simulink model "thermo_simple_with_imc"  (R2017b)
settings: Solver=ode4  StartTime=0.0  StopTime=t_sim  FixedStep=Ts  RelTol=1e-3  EnableMultiTasking=on
undefined symbols (not defined in the file or in its folder): baud, com, D, fTf, fTl, fTt, I, input_fan, input_lamp, input_led, K0, P, reg_output, reg_regulate, reg_request, reg_type, T0, Tf, Ts, Umax, Umin, vstupy, vystupy
libraries: simulink x1, tos_lib x1
settings Model: Creator=tom  LastModifiedBy=www-data
settings DataIOCC: SaveFormat=Array  SignalLoggingSaveFormat=ModelDataLogs  SaveOutput=off  SignalLogging=off  SaveTime=off
settings OptimizationCC: ExpressionDepthLimit=2147483647  LifeSpan=inf
settings DebuggingCC: AlgebraicLoopMsg=none  ArtificialAlgebraicLoopMsg=none  UnderspecifiedInitializationDetection=Classic  MergeDetectMultiDrivingBlocksExec=none  SolverPrmCheckMsg=warning  FcnCallInpInsideContextMsg=warning  StateNameClashWarn=warning  StrictBusMsg=Warning  SFUnexpectedBacktrackingDiag=warning  SFNoUnconditionalDefaultTransitionDiag=warning  SFExecutionAtInitializationDiag=none
settings HardwareCC: ProdBitPerPointer=32  ProdBitPerSizeT=32  ProdBitPerPtrDiffT=32  ProdLargestAtomicFloat=None  ProdIntDivRoundTo=Undefined  ProdEndianess=Unspecified  ProdWordSize=32  ProdHWDeviceType=32-bit Generic
settings ModelReferenceCC: PropagateSignalLabelsOutOfModel=off
settings CodeAppCC: StateflowObjectComments=on
settings GRTTargetCC: TargetLangStandard=C89/C90 (ANSI)  GeneratePreprocessorConditionals=Disable all  CombineOutputUpdateFcns=off  GRTInterface=on
settings ConfigComp: CovMetricSettings=dw  CovHtmlReporting=on  CovSaveCumulativeToWorkspaceVar=on  CovSaveSingleToWorkspaceVar=on  CovExternalEMLEnable=off  CovSFcnEnable=off

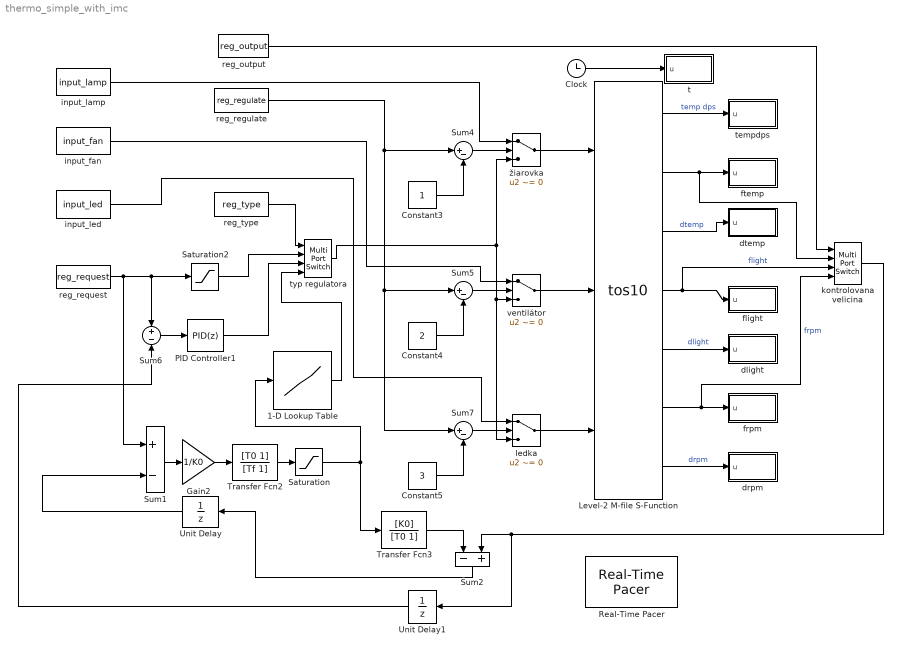
== system thermo_simple_with_imc ==
  1-D Lookup Table : Lookup_n-D  NumberOfTableDimensions=1  BreakpointsForDimension1=vystupy  Table=vstupy  UseLastTableValue=on  InputSameDT=on
  Clock : Clock
  Constant3 : Constant  SampleTime=Ts
  Constant4 : Constant  Value=2  SampleTime=Ts
  Constant5 : Constant  Value=3  SampleTime=Ts
  Gain2 : Gain  Gain=1/K0  SaturateOnIntegerOverflow=on  OutDataTypeStr=Inherit: Same as input  ParamDataTypeStr=Inherit: Same as input
  Level-2 M-file S-Function : M-S-Function  FunctionName=tos10  Parameters=Ts,com,baud,fTt,fTl,fTf
  PID Controller1 : simulink/Continuous/PID Controller  Controller=PID  TimeDomain=Discrete-time  SampleTime=Ts  IntegratorMethod=Forward Euler  FilterMethod=Forward Euler  Form=Parallel  UseFilter=on  ControllerParametersSource=internal  P=P  I=I  D=D  N=10  InitialConditionSource=internal  InitialConditionForIntegrator=0  InitialConditionForFilter=0  ExternalReset=none  LimitOutput=on  UpperSaturationLimit=100  LowerSaturationLimit=0  LinearizeAsGain=off  AntiWindupMode=clamping  Kb=10  TrackingMode=off  Kt=1  PParamMin=[]  PParamMax=[]  IParamMin=[]  IParamMax=[]  DParamMin=[]  DParamMax=[]  NParamMin=[]  NParamMax=[]  KbParamMin=[]  KbParamMax=[]  KtParamMin=[]  KtParamMax=[]  POutMin=[]  POutMax=[]  IOutMin=[]  IOutMax=[]  DOutMin=[]  DOutMax=[]  NOutMin=[]  NOutMax=[]  KbOutMin=[]  KbOutMax=[]  KtOutMin=[]  KtOutMax=[]  IntegratorOutMin=[]  IntegratorOutMax=[]  FilterOutMin=[]  FilterOutMax=[]  SumOutMin=[]  SumOutMax=[]  SumI1OutMin=[]  SumI1OutMax=[]  SumI1OutDataTypeStr=single  SumI2OutMin=[]  SumI2OutMax=[]  SumI3OutMin=[]  SumI3OutMax=[]  SumDOutMin=[]  SumDOutMax=[]  SaturationOutMin=[]  SaturationOutMax=[]  IntegratorContinuousStateAttributes=''  IntegratorStateMustResolveToSignalObject=off  IntegratorRTWStateStorageClass=Auto  FilterContinuousStateAttributes=''  FilterStateMustResolveToSignalObject=off  FilterRTWStateStorageClass=Auto  DifferentiatorICPrevScaledInput=0  DifferentiatorOutMin=[]  DifferentiatorOutMax=[]  InitialConditionSetting=State (most efficient)  FilterDiffOutCoefMin=[]  FilterDiffOutCoefMax=[]  SumDenOutMin=[]  SumDenOutMax=[]  SumNumOutMin=[]  SumNumOutMax=[]  ReciprocalOutMin=[]  ReciprocalOutMax=[]  DivideOutMin=[]  DivideOutMax=[]  TunerSelectOption=Transfer Function Based (PID Tuner App)
  Real-Time Pacer : tos_lib/Real-Time Pacer  simTimePerRealTime=1
  Saturation : Saturate  UpperLimit=Umax  LowerLimit=Umin
  Saturation2 : Saturate  UpperLimit=100  LowerLimit=0  SampleTime=Ts
  Sum1 : Sum  Inputs=+-  SaturateOnIntegerOverflow=on  InputSameDT=on  OutDataTypeStr=Inherit: Same as first input
  Sum2 : Sum  Inputs=-+  SaturateOnIntegerOverflow=on  InputSameDT=on  OutDataTypeStr=Inherit: Same as first input
  Sum4 : Sum  Inputs=|+-  SampleTime=Ts
  Sum5 : Sum  Inputs=|+-  SampleTime=Ts
  Sum6 : Sum  Inputs=+|-  SampleTime=Ts
  Sum7 : Sum  Inputs=|+-  SampleTime=Ts
  Transfer Fcn2 : TransferFcn  Numerator=[T0 1]  Denominator=[Tf 1]
  Transfer Fcn3 : TransferFcn  Numerator=[K0]  Denominator=[T0 1]
  Unit Delay : UnitDelay  SampleTime=-1
  Unit Delay1 : UnitDelay  SampleTime=Ts
  dlight : MATLAB Function  TreatAsAtomicUnit=on  SystemSampleTime=Ts
  drpm : MATLAB Function  TreatAsAtomicUnit=on  SystemSampleTime=Ts
  dtemp : MATLAB Function  TreatAsAtomicUnit=on  SystemSampleTime=Ts
  flight : MATLAB Function  TreatAsAtomicUnit=on  SystemSampleTime=Ts
  frpm : MATLAB Function  TreatAsAtomicUnit=on  SystemSampleTime=Ts
  ftemp : MATLAB Function  TreatAsAtomicUnit=on  SystemSampleTime=Ts
  input_fan : Constant  Value=input_fan  SampleTime=Ts
  input_lamp : Constant  Value=input_lamp  SampleTime=Ts
  input_led : Constant  Value=input_led  SampleTime=Ts
  kontrolovana velicina : MultiPortSwitch  OutDataTypeStr=double  SampleTime=Ts
  ledka : Switch  Criteria=u2 ~= 0  OutDataTypeStr=double
  reg_output : Constant  Value=reg_output  SampleTime=Ts
  reg_regulate : Constant  Value=reg_regulate  SampleTime=Ts
  reg_request : Constant  Value=reg_request  SampleTime=Ts
  reg_type : Constant  Value=reg_type  SampleTime=Ts
  t : MATLAB Function  TreatAsAtomicUnit=on  SystemSampleTime=Ts
  tempdps : MATLAB Function  TreatAsAtomicUnit=on  SystemSampleTime=Ts
  typ regulatora : MultiPortSwitch  OutDataTypeStr=double  SampleTime=Ts
  ventilátor : Switch  Criteria=u2 ~= 0  OutDataTypeStr=double
  žiarovka : Switch  Criteria=u2 ~= 0  OutDataTypeStr=double
  wires:
  ledka/1 -> Level-2 M-file S-Function/3
  Level-2 M-file S-Function/7 -> drpm/1(u)  "drpm"
  Sum4/1 -> žiarovka/2
  input_fan/1 -> ventilátor/1
  reg_regulate/1 -> Sum7/1, Sum5/1, Sum4/1
  Saturation2/1 -> typ regulatora/2
  Sum6/1 -> PID Controller1/1
  Level-2 M-file S-Function/1 -> tempdps/1(u)  "temp dps"
  Level-2 M-file S-Function/5 -> dlight/1(u)  "dlight"
  PID Controller1/1 -> typ regulatora/3
  žiarovka/1 -> Level-2 M-file S-Function/1
  ventilátor/1 -> Level-2 M-file S-Function/2
  reg_request/1 -> Sum1/1, Sum6/1, Saturation2/1
  Unit Delay1/1 -> Sum6/2
  Level-2 M-file S-Function/3 -> dtemp/1(u)  "dtemp"
  Constant4/1 -> Sum5/2
  Level-2 M-file S-Function/4 -> kontrolovana velicina/3, flight/1(u)  "flight"
  Level-2 M-file S-Function/6 -> kontrolovana velicina/4, frpm/1(u)  "frpm"
  Constant3/1 -> Sum4/2
  typ regulatora/1 -> žiarovka/3, ventilátor/3, ledka/3
  Clock/1 -> t/1(u)
  input_lamp/1 -> žiarovka/1
  reg_output/1 -> kontrolovana velicina/1
  Sum5/1 -> ventilátor/2
  Constant5/1 -> Sum7/2
  reg_type/1 -> typ regulatora/1
  kontrolovana velicina/1 -> Sum2/2, Unit Delay1/1
  Level-2 M-file S-Function/2 -> kontrolovana velicina/2, ftemp/1(u)
  Sum7/1 -> ledka/2
  input_led/1 -> ledka/1
  Saturation/1 -> 1-D Lookup Table/1, Transfer Fcn3/1
  Gain2/1 -> Transfer Fcn2/1
  Sum1/1 -> Gain2/1
  Transfer Fcn2/1 -> Saturation/1
  Transfer Fcn3/1 -> Sum2/1
  Unit Delay/1 -> Sum1/2
  Sum2/1 -> Unit Delay/1
  1-D Lookup Table/1 -> typ regulatora/4

== matlab function thermo_simple_with_imc/ftemp ==
  data: u input
function fcn(u)
%#eml
eml.extrinsic('num2str');
eml.extrinsic('strcat');
eml.extrinsic('evalin');
evalin('base',strcat('ftemp(end+1)=', num2str(u),';'));
end

== matlab function thermo_simple_with_imc/tempdps ==
  data: u input
function fcn(u)
%#eml
eml.extrinsic('num2str');
eml.extrinsic('strcat');
eml.extrinsic('evalin');
evalin('base',strcat('tempdps(end+1)=', num2str(u),';'));
end

== matlab function thermo_simple_with_imc/dtemp ==
  data: u input
function fcn(u)
%#eml
eml.extrinsic('num2str');
eml.extrinsic('strcat');
eml.extrinsic('evalin');
evalin('base',strcat('dtemp(end+1)=', num2str(u),';'));
end

== matlab function thermo_simple_with_imc/frpm ==
  data: u input
function fcn(u)
%#eml
eml.extrinsic('num2str');
eml.extrinsic('strcat');
eml.extrinsic('evalin');
evalin('base',strcat('frpm(end+1)=', num2str(u),';'));
end

== matlab function thermo_simple_with_imc/drpm ==
  data: u input
function fcn(u)
%#eml
eml.extrinsic('num2str');
eml.extrinsic('strcat');
eml.extrinsic('evalin');
evalin('base',strcat('drpm(end+1)=', num2str(u),';'));
end

== matlab function thermo_simple_with_imc/flight ==
  data: u input
function fcn(u)
%#eml
eml.extrinsic('num2str');
eml.extrinsic('strcat');
eml.extrinsic('evalin');
evalin('base',strcat('flight(end+1)=', num2str(u),';'));
end

== matlab function thermo_simple_with_imc/dlight ==
  data: u input
function fcn(u)
%#eml
eml.extrinsic('num2str');
eml.extrinsic('strcat');
eml.extrinsic('evalin');
evalin('base',strcat('dlight(end+1)=', num2str(u),';'));
end

== matlab function thermo_simple_with_imc/t ==
  data: u input
function fcn(u)
%#eml
eml.extrinsic('num2str');
eml.extrinsic('strcat');
eml.extrinsic('evalin');
evalin('base',strcat('t(end+1)=', num2str(u),';'));
end
